simulink subsystem "EncoderAJdis"  (R2023b)
settings: Solver=VariableStepAuto  StartTime=0.0  StopTime=10.0  RelTol=1e-3
libraries: arduinosensorlib x2
settings Model: Creator=johan  LastModifiedBy=johan

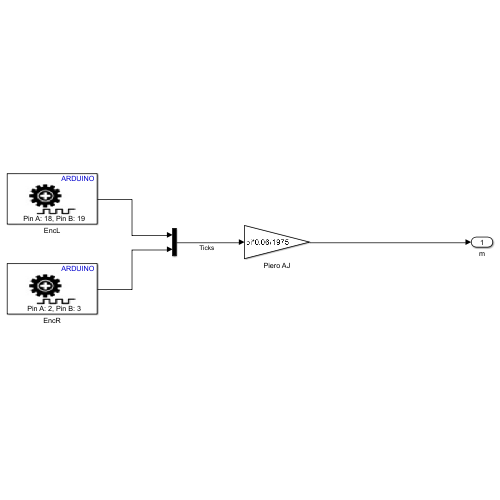
[thumbnail: Simulink's stored preview of the top-level diagram]
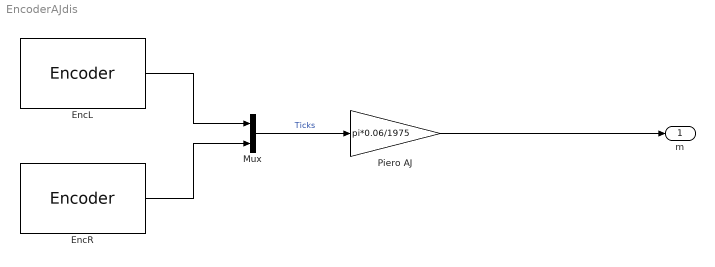
== system EncoderAJdis ==
  EncL : arduinosensorlib/Encoder  InputA=18  InputB=19  Mode=No reset  SampleTime=-1
  EncR : arduinosensorlib/Encoder  InputA=2  InputB=3  Mode=No reset  SampleTime=-1
  Mux : Mux  Inputs=2
  Piero AJ : Gain  Gain=pi*0.06/1975
  m : Outport
  wires:
  Piero AJ/1 -> m/1
  EncR/1 -> Mux/2
  EncL/1 -> Mux/1
  Mux/1 -> Piero AJ/1  "Ticks"
